simulink model "jointSpaceInverseDynamicsControl"  (R2021a)
settings: Solver=VariableStepAuto  StartTime=0.0  StopTime=1  RelTol=1e-3
values from neighbouring files (symbols this model uses):
  Kd = diag([40, 30, 40])    [assignment7_main.m]
  Kp = diag([300, 200, 300])    [assignment7_main.m]
  q_d_const = [0.1 ... (first row only)    [assignment7_main.m]
libraries: vrlib x1, robotcorelib x1
settings Model: Creator=fabio  LastModifiedBy=fabio

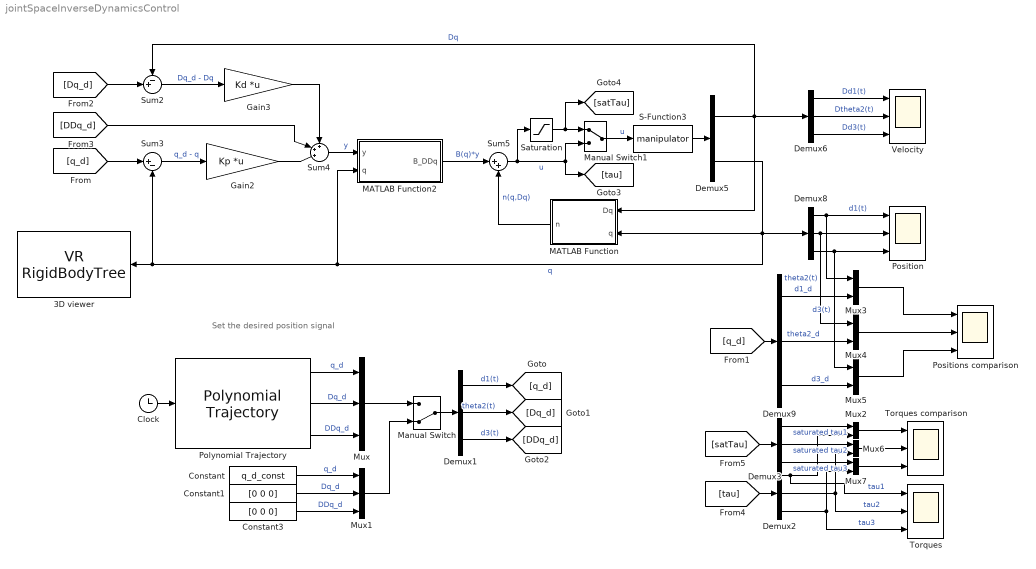
== system jointSpaceInverseDynamicsControl ==
  note: Set the desired position signal
  3D viewer : vrlib/VR RigidBodyTree  RBT=robot  useRBT=off  Ts=0.5  ForceViewerOpen=on
      settings: SourceProductBaseCode=SL
  Clock : Clock
  Constant : Constant  Value=q_d_const
  Constant1 : Constant  Value=[0 0 0]
  Constant3 : Constant  Value=[0 0 0]
  Demux{1..3,6,8..9} (6 alike) : Demux  Outputs=3
  Demux5 : Demux  Outputs=[3 3]
  Gain2 : Gain  Gain=Kp  Multiplication=Matrix(K*u) (u vector)
  Gain3 : Gain  Gain=Kd  Multiplication=Matrix(K*u) (u vector)
  MATLAB Function : MATLAB Function  TreatAsAtomicUnit=on
  MATLAB Function2 : MATLAB Function  TreatAsAtomicUnit=on
  Manual Switch : ManualSwitch  CurrentSetting=0
  Manual Switch1 : ManualSwitch
  Mux : Mux  Inputs=3
  Mux1 : Mux  Inputs=3
  Mux{2..7} (6 alike) : Mux  Inputs=2
  Polynomial Trajectory : robotcorelib/Polynomial Trajectory  WaypointSource=Internal  Waypoints=q_d  TimePoints=[ 0, 1, 2]  TimeInterval=[ 1, 4 ]  Method=Cubic Polynomial  ParameterSource=Internal  VelocityBoundaryCondition=zeros( 3, 3 )  AccelerationBoundaryCondition=zeros( 2, 5 )  SimulateUsing=Interpreted execution
  Position : Scope  NumInputPorts=3
  Positions comparison : Scope  NumInputPorts=3
  S-Function3 : S-Function  FunctionName=manipulator  Parameters=myRobot  SFunctionDeploymentMode=off  EnableBusSupport=off
  Saturation : Saturate  UpperLimit=20  LowerLimit=-20
  Sum2 : Sum  Inputs=-+|
  Sum3 : Sum  Inputs=|+-
  Sum4 : Sum  Inputs=+++|
  Sum5 : Sum  Inputs=|++
  Torques : Scope  NumInputPorts=3
  Torques comparison : Scope  NumInputPorts=3
  Velocity : Scope  NumInputPorts=3
  wires:
  Demux9/2 -> Mux4/2  "theta2_d"
  Mux4/1 -> Positions comparison/2
  Mux3/1 -> Positions comparison/1
  Manual Switch1/1 -> S-Function3/1  "u"
  Demux9/3 -> Mux5/2  "d3_d"
  Sum3/1 -> Gain2/1  "q_d - q"
  Demux9/1 -> Mux3/2  "d1_d"
  Demux8/2 -> Position/2, Mux4/1  "theta2(t)"
  Demux8/3 -> Position/3, Mux5/1  "d3(t)"
  Demux6/3 -> Velocity/3  "Dd3(t)"
  Demux6/2 -> Velocity/2  "Dtheta2(t)"
  Demux6/1 -> Velocity/1  "Dd1(t)"
  S-Function3/1 -> Demux5/1
  Demux8/1 -> Position/1, Mux3/1  "d1(t)"
  Mux5/1 -> Positions comparison/3
  Demux5/1 -> MATLAB Function/1(Dq), Demux6/1, Sum2/1  "Dq"
  Gain2/1 -> Sum4/3
  Sum2/1 -> Gain3/1  "Dq_d - Dq"
  Gain3/1 -> Sum4/1
  Sum4/1 -> MATLAB Function2/1(y)  "y"
  MATLAB Function2/1(B_DDq) -> Sum5/1  "B(q)*y"
  MATLAB Function/1(n) -> Sum5/2  "n(q,Dq)"
  Clock/1 -> Polynomial Trajectory/1
  Polynomial Trajectory/2 -> Mux/2  "Dq_d"
  [DDq_d] -> Sum4/2
  [q_d] -> Sum3/1
  [Dq_d] -> Sum2/2
  [q_d] -> Demux9/1
  Polynomial Trajectory/1 -> Mux/1  "q_d"
  Polynomial Trajectory/3 -> Mux/3  "DDq_d"
  Mux/1 -> Manual Switch/1
  Manual Switch/1 -> Demux1/1
  Demux1/1 -> [q_d]  "d1(t)"
  Demux1/2 -> [Dq_d]  "theta2(t)"
  Demux1/3 -> [DDq_d]  "d3(t)"
  Constant/1 -> Mux1/1  "q_d"
  Constant1/1 -> Mux1/2  "Dq_d"
  Mux1/1 -> Manual Switch/2
  Constant3/1 -> Mux1/3  "DDq_d"
  Demux2/1 -> Torques/1, Mux2/2  "tau1"
  [tau] -> Demux2/1
  Saturation/1 -> [satTau], Manual Switch1/1
  [satTau] -> Demux3/1
  Demux3/1 -> Mux2/1  "saturated tau1"
  Mux2/1 -> Torques comparison/1
  Mux6/1 -> Torques comparison/2
  Mux7/1 -> Torques comparison/3
  Demux2/2 -> Torques/2, Mux6/2  "tau2"
  Demux3/2 -> Mux6/1  "saturated tau2"
  Demux3/3 -> Mux7/1  "saturated tau3"
  Demux2/3 -> Torques/3, Mux7/2  "tau3"
  Sum5/1 -> Manual Switch1/2, [tau], Saturation/1  "u"
  Demux5/2 -> Demux8/1, MATLAB Function/2(q), MATLAB Function2/2(q), Sum3/2, 3D viewer/1  "q"

== matlab function jointSpaceInverseDynamicsControl/MATLAB Function2 ==
  data: y input; B_DDq output; q input
function B_DDq = B_q(y,q)
    B_DDq = get_B_matrix(q)*y;
end

== matlab function jointSpaceInverseDynamicsControl/MATLAB Function ==
  data: Dq input; n output; q input
function n = n_q_Dq(Dq, q)
    
    %To get the "perfect" matrices use the following code
    C = get_C_matrix(q,Dq);
    G = get_G_matrix(q);
    
    
    %To get the "wrongly estimated" matrices use the following code   
%     theta2 = q(2);   d3 = q(3); 
%     Dtheta2 = Dq(2); Dd3 = Dq(3); 
%     
%     m_Link4 = 0.16;  %0.2kg is the correct value
% 
%     C = [0,                         0,                        0;
%          0,            m_Link4*Dd3*d3,       m_Link4*Dtheta2*d3;
%          0,       -m_Link4*Dtheta2*d3,                        0];
%    
%     G = [           0                           ;
%          -(981*m_Link4*sin(theta2)*d3)/100 ;
%           (981*m_Link4*cos(theta2))/100    ];


    
    n = C*Dq + G; %F = friction is neglected

end
